simulink model "thermoguard_realistic_simscape"  (R2026a)
settings: Solver=VariableStepAuto  StopTime=2000  AbsTol=1e-3
undefined symbols (not defined in the file or in its folder): T_a, T_e0
libraries: fl_lib x18, nesl_utility x6
settings Model: Creator=xerxes  LastModifiedBy=xerxes
settings DebuggingCC: SymbolicDimsDataTypeCodeGenerationDiagnostic=none

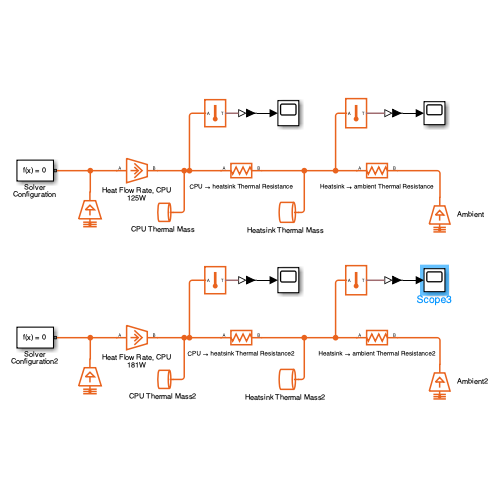
[thumbnail: Simulink's stored preview of the top-level diagram]
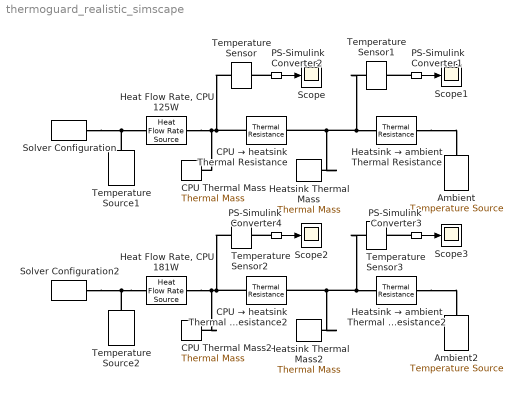
== system thermoguard_realistic_simscape ==
  Ambient : fl_lib/Thermal/Thermal Sources/Temperature Source  temperature=T_a degC
  Ambient2 : fl_lib/Thermal/Thermal Sources/Temperature Source  temperature=T_a degC
  CPU Thermal Mass : fl_lib/Thermal/Thermal Elements/Thermal Mass  mass_type=foundation.enum.constant_variable.constant  mass=m_cpu kg  sp_heat=cp_cpu J/(K*kg)  mass_min=1e-6 kg  num_ports=foundation.enum.numPorts2.one  m_specify=off  m_priority=High  m=1 kg  m_nominal_specify=off  m_nominal_value=1  m_nominal_unit=kg  T_specify=on  T_priority=High  T=T_e0 degC  T_nominal_specify=off  T_nominal_value=1  T_nominal_unit=K  Q_specify=off  Q_priority=None  Q=0 W  Q_nominal_specify=off  Q_nominal_value=1  Q_nominal_unit=W
  CPU Thermal Mass2 : fl_lib/Thermal/Thermal Elements/Thermal Mass  mass_type=foundation.enum.constant_variable.constant  mass=m_cpu kg  sp_heat=cp_cpu J/(K*kg)  mass_min=1e-6 kg  num_ports=foundation.enum.numPorts2.one  m_specify=off  m_priority=High  m=1 kg  m_nominal_specify=off  m_nominal_value=1  m_nominal_unit=kg  T_specify=on  T_priority=High  T=T_a degC  T_nominal_specify=off  T_nominal_value=1  T_nominal_unit=K  Q_specify=off  Q_priority=None  Q=0 W  Q_nominal_specify=off  Q_nominal_value=1  Q_nominal_unit=W
  CPU → heatsink Thermal Resistance : fl_lib/Thermal/Thermal Elements/Thermal Resistance  resistance=R_eh K/W  T_specify=off  T_priority=None  T=0 K  T_nominal_specify=off  T_nominal_value=1  T_nominal_unit=K  Q_specify=off  Q_priority=None  Q=0 W  Q_nominal_specify=off  Q_nominal_value=1  Q_nominal_unit=W
  CPU → heatsink Thermal Resistance2 : fl_lib/Thermal/Thermal Elements/Thermal Resistance  resistance=R_eh K/W  T_specify=off  T_priority=None  T=0 K  T_nominal_specify=off  T_nominal_value=1  T_nominal_unit=K  Q_specify=off  Q_priority=None  Q=0 W  Q_nominal_specify=off  Q_nominal_value=1  Q_nominal_unit=W
  "Heat Flow Rate, CPU 125W" : fl_lib/Thermal/Thermal Sources/Heat Flow Rate Source  heat_flow=125 W
  "Heat Flow Rate, CPU 181W" : fl_lib/Thermal/Thermal Sources/Heat Flow Rate Source  heat_flow=181 W
  Heatsink Thermal Mass : fl_lib/Thermal/Thermal Elements/Thermal Mass  mass_type=foundation.enum.constant_variable.constant  mass=m_heatsink kg  sp_heat=cp_heatsink J/(K*kg)  mass_min=1e-6 kg  num_ports=foundation.enum.numPorts2.one  m_specify=off  m_priority=High  m=1 kg  m_nominal_specify=off  m_nominal_value=1  m_nominal_unit=kg  T_specify=on  T_priority=High  T=T_a degC  T_nominal_specify=off  T_nominal_value=1  T_nominal_unit=K  Q_specify=off  Q_priority=None  Q=0 W  Q_nominal_specify=off  Q_nominal_value=1  Q_nominal_unit=W
  Heatsink Thermal Mass2 : fl_lib/Thermal/Thermal Elements/Thermal Mass  mass_type=foundation.enum.constant_variable.constant  mass=m_heatsink kg  sp_heat=cp_heatsink J/(K*kg)  mass_min=1e-6 kg  num_ports=foundation.enum.numPorts2.one  m_specify=off  m_priority=High  m=1 kg  m_nominal_specify=off  m_nominal_value=1  m_nominal_unit=kg  T_specify=on  T_priority=High  T=T_a degC  T_nominal_specify=off  T_nominal_value=1  T_nominal_unit=K  Q_specify=off  Q_priority=None  Q=0 W  Q_nominal_specify=off  Q_nominal_value=1  Q_nominal_unit=W
  Heatsink → ambient Thermal Resistance : fl_lib/Thermal/Thermal Elements/Thermal Resistance  resistance=R_ha_maxfan K/W  T_specify=off  T_priority=None  T=0 K  T_nominal_specify=off  T_nominal_value=1  T_nominal_unit=K  Q_specify=off  Q_priority=None  Q=0 W  Q_nominal_specify=off  Q_nominal_value=1  Q_nominal_unit=W
  Heatsink → ambient Thermal Resistance2 : fl_lib/Thermal/Thermal Elements/Thermal Resistance  resistance=R_ha_maxfan K/W  T_specify=off  T_priority=None  T=0 K  T_nominal_specify=off  T_nominal_value=1  T_nominal_unit=K  Q_specify=off  Q_priority=None  Q=0 W  Q_nominal_specify=off  Q_nominal_value=1  Q_nominal_unit=W
  PS-Simulink Converter{1..4} (4 alike) : nesl_utility/PS-Simulink Converter  PhysicalDomain=network_engine_domain  SubClassName=ps_output  LeftPortType=input  RightPortType=output  PseudoPeriodic=off  Frequencies=[]  VectorFormat=inherit  Unit=degC  AffineConversion=on
  Scope{,1..3} (4 alike) : Scope
      Scope settings: ActiveDisplayYMinimum=20.156250000000441  ActiveDisplayYMaximum=68.593749999996035
      Scope1 settings: ActiveDisplayYMinimum=20.791750000000967  ActiveDisplayYMaximum=62.874249999991292
      Scope2 settings: ActiveDisplayYMinimum=17.986250000001  ActiveDisplayYMaximum=88.123749999990991  DataLoggingVariableName=ScopeData2
      Scope3 settings: ActiveDisplayYMinimum=20.791750000000967  ActiveDisplayYMaximum=62.874249999991292  DataLoggingVariableName=ScopeData3
  Solver Configuration : nesl_utility/Solver Configuration  PhysicalDomain=network_engine_domain  SubClassName=solver  LeftPortType=input  RightPortType=generic  Tones=[]  Harmonics=[]  SimulateNoise=off  Profile=off  UseLocalSampling=off  EnableSwitchedLinearOptims=on  FrequencyDomain=off  UseCCode=off  RelTol=0.001  AbsTol=0.001  MinStep=1e-09  ToWorkspace=off  RevertToSquareIcSolve=off  NumHomotopyIterations=100  PhasorMode=off  PhasorModeNumHarmonics=1  ConsistencySolver=NEWTON_XTOL_AFTER_FTOL  CanonicalOrdering=CANONICAL  OptimizeIntermediates=UNOPTIMIZED  IndexReductionMethod=DerivativeReplacement  DoDC=off  ResidualTolerance=1e-09  ConsistencyTolSource=GLOBAL  ConsistencyAbsTol=0.001  ConsistencyRelTol=0.001  ConsistencyTolFactor=0.001  UseLocalSolver=off  LocalSolverChoice=NE_BACKWARD_EULER_ADVANCER  ResolveIndetEquations=on  FunctionEvalNumThread=1  LocalSolverSampleTime=0.001  DoFixedCost=off  MaxNonlinIter=3  MaxModeIter=2  ComputeImpulses=off  ImpulseIterations=2  LinearAlgebra=auto  LinearAlgebraNumThread=0  EquationFormulation=NE_TIME_EF  DelaysMemoryBudget=1024  AutomaticFiltering=on  FilteringTimeConstant=0.001  PartitionStorageMethod=AS_NEEDED  PartitionMemoryBudget=1024  PartitionMethod=ROBUST  MultibodyUseLocalSolver=off  MultibodyLocalSolverChoice=ODE1  MultibodyLocalSolverSampleTime=0.001
  Solver Configuration2 : nesl_utility/Solver Configuration  PhysicalDomain=network_engine_domain  SubClassName=solver  LeftPortType=input  RightPortType=generic  Tones=[]  Harmonics=[]  SimulateNoise=off  Profile=off  UseLocalSampling=off  EnableSwitchedLinearOptims=on  FrequencyDomain=off  UseCCode=off  RelTol=0.001  AbsTol=0.001  MinStep=1e-09  ToWorkspace=off  RevertToSquareIcSolve=off  NumHomotopyIterations=100  PhasorMode=off  PhasorModeNumHarmonics=1  ConsistencySolver=NEWTON_XTOL_AFTER_FTOL  CanonicalOrdering=CANONICAL  OptimizeIntermediates=UNOPTIMIZED  IndexReductionMethod=DerivativeReplacement  DoDC=off  ResidualTolerance=1e-09  ConsistencyTolSource=GLOBAL  ConsistencyAbsTol=0.001  ConsistencyRelTol=0.001  ConsistencyTolFactor=0.001  UseLocalSolver=off  LocalSolverChoice=NE_BACKWARD_EULER_ADVANCER  ResolveIndetEquations=on  FunctionEvalNumThread=1  LocalSolverSampleTime=0.001  DoFixedCost=off  MaxNonlinIter=3  MaxModeIter=2  ComputeImpulses=off  ImpulseIterations=2  LinearAlgebra=auto  LinearAlgebraNumThread=0  EquationFormulation=NE_TIME_EF  DelaysMemoryBudget=1024  AutomaticFiltering=on  FilteringTimeConstant=0.001  PartitionStorageMethod=AS_NEEDED  PartitionMemoryBudget=1024  PartitionMethod=ROBUST  MultibodyUseLocalSolver=off  MultibodyLocalSolverChoice=ODE1  MultibodyLocalSolverSampleTime=0.001
  Temperature Sensor{,1..3} (4 alike) : fl_lib/Thermal/Thermal Sensors/Temperature Sensor  temperature_measure=foundation.enum.MeasurementReference.absolute
  Temperature Source1 : fl_lib/Thermal/Thermal Sources/Temperature Source  temperature=T_a degC
  Temperature Source2 : fl_lib/Thermal/Thermal Sources/Temperature Source  temperature=T_a degC
  wires:
  PS-Simulink Converter2/1 -> Scope/1
  PS-Simulink Converter1/1 -> Scope1/1
  PS-Simulink Converter4/1 -> Scope2/1
  PS-Simulink Converter3/1 -> Scope3/1
  connections:
  PS-Simulink Converter2/LConn1 -- Temperature Sensor/RConn1
  Temperature Sensor/LConn1 -- CPU → heatsink Thermal Resistance/LConn1 -- "Heat Flow Rate, CPU 125W"/LConn1 -- CPU Thermal Mass/LConn1
  Heatsink Thermal Mass/LConn1 -- Temperature Sensor1/LConn1 -- Heatsink → ambient Thermal Resistance/LConn1 -- CPU → heatsink Thermal Resistance/RConn1
  Heatsink → ambient Thermal Resistance/RConn1 -- Ambient/LConn1
  Temperature Source1/LConn1 -- Solver Configuration/RConn1 -- "Heat Flow Rate, CPU 125W"/RConn1
  PS-Simulink Converter1/LConn1 -- Temperature Sensor1/RConn1
  "Heat Flow Rate, CPU 181W"/RConn1 -- Solver Configuration2/RConn1 -- Temperature Source2/LConn1
  CPU Thermal Mass2/LConn1 -- "Heat Flow Rate, CPU 181W"/LConn1 -- Temperature Sensor2/LConn1 -- CPU → heatsink Thermal Resistance2/LConn1
  Heatsink Thermal Mass2/LConn1 -- Temperature Sensor3/LConn1 -- Heatsink → ambient Thermal Resistance2/LConn1 -- CPU → heatsink Thermal Resistance2/RConn1
  PS-Simulink Converter3/LConn1 -- Temperature Sensor3/RConn1
  PS-Simulink Converter4/LConn1 -- Temperature Sensor2/RConn1
  Heatsink → ambient Thermal Resistance2/RConn1 -- Ambient2/LConn1
